simulink model "integrator_anti_windup_order_model"  (R2018b)
settings: Solver=ode45  StartTime=0.0  StopTime=10.0  RelTol=1e-3  EnableMultiTasking=on
values from neighbouring files (symbols this model uses):
  integrator_lower_limit = -4    [MAIN_integrator_anti_windup_order.m]
  integrator_upper_limit = 4    [MAIN_integrator_anti_windup_order.m]
  KI = 2    [MAIN_integrator_anti_windup_order.m]
  step_duration = 2    [MAIN_integrator_anti_windup_order.m]
  step_magnitude = 5    [MAIN_integrator_anti_windup_order.m]
  step_time = 5    [MAIN_integrator_anti_windup_order.m]
settings Model: Creator=lum  LastModifiedBy=Christopher
settings DataIOCC: LimitDataPoints=on  SaveFormat=Array  SignalLoggingSaveFormat=ModelDataLogs
settings OptimizationCC: ExpressionDepthLimit=2147483647  LifeSpan=inf
settings DebuggingCC: UnderspecifiedInitializationDetection=Classic  MergeDetectMultiDrivingBlocksExec=none  SolverPrmCheckMsg=warning  FcnCallInpInsideContextMsg=warning  StateNameClashWarn=warning  SFUnexpectedBacktrackingDiag=warning  SFNoUnconditionalDefaultTransitionDiag=warning  SFExecutionAtInitializationDiag=none
settings HardwareCC: ProdBitPerPointer=32  ProdBitPerSizeT=32  ProdBitPerPtrDiffT=32  ProdLargestAtomicFloat=None  ProdIntDivRoundTo=Undefined  ProdEndianess=Unspecified  ProdWordSize=32  ProdHWDeviceType=32-bit Generic
settings ModelReferenceCC: PropagateSignalLabelsOutOfModel=off
settings SFSimCC: SimUseLocalCustomCode=off
settings RTWCC: RTWUseLocalCustomCode=off
settings CodeAppCC: StateflowObjectComments=on
settings GRTTargetCC: TargetLangStandard=C89/C90 (ANSI)  GeneratePreprocessorConditionals=Disable all  CombineOutputUpdateFcns=off  GRTInterface=on
settings ConfigComp: CovMetricSettings=dw  CovHtmlReporting=on  CovSaveCumulativeToWorkspaceVar=on  CovSaveSingleToWorkspaceVar=on  CovExternalEMLEnable=off

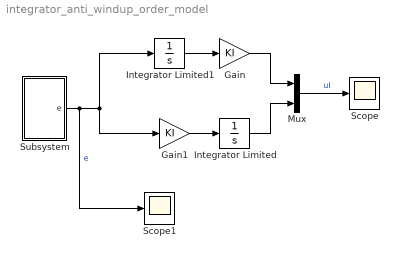
== system integrator_anti_windup_order_model ==
  Gain : Gain  Gain=KI
  Gain1 : Gain  Gain=KI
  Integrator Limited : Integrator  LimitOutput=on  UpperSaturationLimit=integrator_upper_limit  LowerSaturationLimit=integrator_lower_limit
  Integrator Limited1 : Integrator  LimitOutput=on  UpperSaturationLimit=integrator_upper_limit  LowerSaturationLimit=integrator_lower_limit
  Mux : Mux  Inputs=2
  Scope : Scope
  Scope1 : Scope
  Subsystem : Subsystem
  wires:
  Subsystem/1(e) -> Integrator Limited1/1, Gain1/1, Scope1/1  "e"
  Integrator Limited/1 -> Mux/2
  Mux/1 -> Scope/1  "uI"
  Integrator Limited1/1 -> Gain/1
  Gain/1 -> Mux/1
  Gain1/1 -> Integrator Limited/1

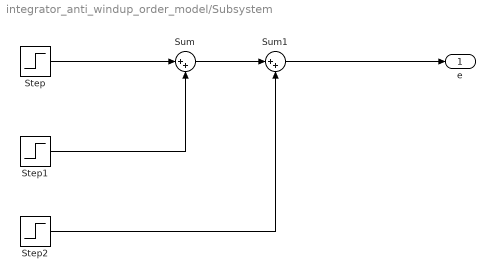
== system integrator_anti_windup_order_model/Subsystem ==
  Step : Step  Time=step_time  After=step_magnitude  SampleTime=0
  Step1 : Step  Time=step_time + step_duration  After=-2*step_magnitude  SampleTime=0
  Step2 : Step  Time=step_time + 2*step_duration  After=step_magnitude  SampleTime=0
  Sum : Sum  Inputs=|++
  Sum1 : Sum  Inputs=|++
  e : Outport
  wires:
  Step/1 -> Sum/1
  Step1/1 -> Sum/2
  Sum/1 -> Sum1/1
  Step2/1 -> Sum1/2
  Sum1/1 -> e/1
